simulink subsystem "IR_LED_Pattern"  (R2024a)
settings: Solver=VariableStepAuto  StartTime=0.0  StopTime=10.0  RelTol=1e-3
settings Model: Creator=JesseJabezArendse  LastModifiedBy=griff
settings RTWCC: GPUComputeCapability=3.5

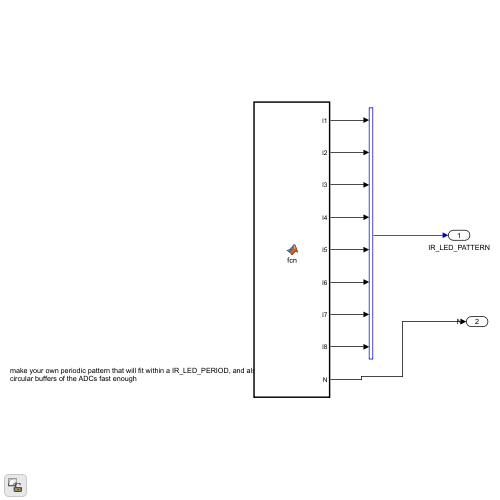
[thumbnail: Simulink's stored preview of the top-level diagram]
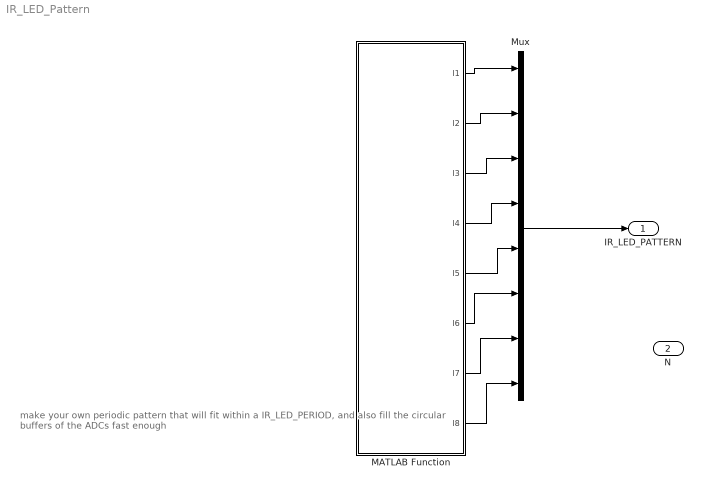
== system IR_LED_Pattern ==
  note: make your own periodic pattern that will fit within a IR_LED_PERIOD, and also fill the circular buffers of the ADCs fast enough
  MATLAB Function : MATLAB Function  TreatAsAtomicUnit=on
  Mux : Mux  Inputs=8
  IR_LED_PATTERN : Outport
  N : Outport  Port=2
  wires:
  Mux/1 -> IR_LED_PATTERN/1
  MATLAB Function/1(l1) -> Mux/1
  MATLAB Function/2(l2) -> Mux/2
  MATLAB Function/3(l3) -> Mux/3
  MATLAB Function/4(l4) -> Mux/4
  MATLAB Function/5(l5) -> Mux/5
  MATLAB Function/6(l6) -> Mux/6
  MATLAB Function/7(l7) -> Mux/7
  MATLAB Function/8(l8) -> Mux/8
  ? -> N/1

== matlab function IR_LED_Pattern/MATLAB Function ==
  data: l1 output; l2 output; l3 output; l4 output; l5 output; l6 output; l7 output; l8 output
function [l1,l2,l3,l4,l5,l6,l7,l8] = fcn()

persistent c 
if isempty(c)
    c=0;
end
c= c+1;
result=[1,0,0,0,0,0,0,0];
result = circshift(result,c);
l1=result(1);
l2=result(3);
l3=result(5);
l4=result(7);
l5=result(7);
l6=result(5);
l7=result(3);
l8=result(1);




end
